simulink model "webserver_start_firstpage_demo"  (Simulink 7.3)
settings: Solver=FixedStepDiscrete  SolverMode=SingleTasking  StartTime=0.0  StopTime=10.0  RelTol=1e-3
PreLoadFcn:
  | waijung.modelPreload; % Required for working with Waijung Blockset. Do not remove.
undefined symbols (not defined in the file): A1, A2, A7, B13, C1, C4, C5, G11, G13, HSEOSC, Link, LQFP144, ST, STM32F429ZI
libraries: waijung_webserver x3, stm32f4_adc_lib x1, stm32f4_io_lib x1, stm32f4_device_config_lib x1
CloseFcn:
  | waijung.modelClose; % Required for working with Waijung Blockset. Do not remove.
settings Model: Creator=Krisada  LastModifiedBy=Krisada
settings OptimizationCC: InlineParams=on  OptimizeModelRefInitCode=on  LifeSpan=1
settings HardwareCC: ProdEndianess=LittleEndian  ProdHWDeviceType=ARM Compatible->Cortex - M4  TargetEndianess=LittleEndian  TargetHWDeviceType=ARM Compatible->Cortex - M4
settings RTWCC: SystemTargetFile=stm32f4.tlc  GenerateMakefile=off  TemplateMakefile=ert_default_tmf  Description=STM32F4 Target  ProcessScript=stm32f4_make_rtw_hook
settings CodeAppCC: IgnoreCustomStorageClasses=off
settings STFCustomTargetCC: ModelReferenceCompliant=off  CombineOutputUpdateFcns=on  ERTCustomFileBanners=on  SupportContinuousTime=off  SupportNonInlinedSFcns=off  SystemTargetFile=stm32f4.tlc
settings ERTTargetCC: MultiwordLength=2048  ModelReferenceCompliant=off  ParMdlRefBuildCompliant=off  CompOptLevelCompliant=off  ERTFirstTimeCompliant=off  ModelStepFunctionPrototypeControlCompliant=off  CPPClassGenCompliant=off  ExtModeMexFile=noextcomm  InlinedParameterPlacement=NonHierarchical  ERTSrcFileBannerTemplate=stm32f4_code_template.cgt  ERTHdrFileBannerTemplate=stm32f4_code_template.cgt  ERTDataSrcFileTemplate=stm32f4_code_template.cgt  ERTDataHdrFileTemplate=stm32f4_code_template.cgt  ERTCustomFileTemplate=stm32f4_file_process.tlc

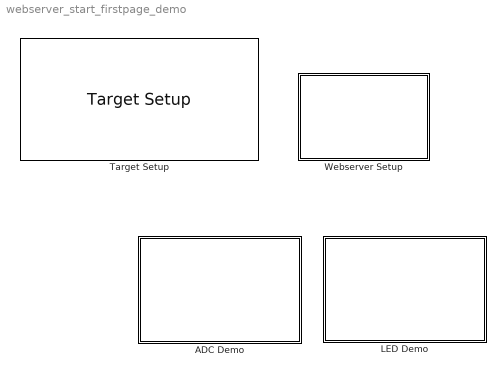
== system webserver_start_firstpage_demo ==
  ADC Demo : Subsystem
  LED Demo : Subsystem
  Target Setup : stm32f4_device_config_lib/Target Setup  Priority=100  compiler=GNU ARM  previous_compiler=GNU ARM  mcu=STM32F429ZI (LQFP144)  mcustr=STM32F429ZI  clockconfig=HSEOSC-8MHz  system_stm32f4xx_c_path=F:\trunk\targets\stm32f4_target\stm32f4\utils\system_stm32f4xx_default\STM32F429_439xx\hseosc8mhz  showmemoryconfiguration=on  stacksize=0x2000  heapsize=0x2000  enableautocompiledownload=on  fullchiperase=on  programmerinterface=ST-Link  editctrlstr=on  compilercontrolstr=$(patsubst %, -I%, .) -mcpu=cortex-m4 -mthumb -mthumb-interwork -mfloat-abi=hard -mfpu=fpv4-sp-d16 -ffast-math -Wall -Wextra -Ofast  assemblercontrolstr=$(patsubst %, -I%, .) -mcpu=cortex-m4 -mthumb -mthumb-interwork -mfloat-abi=hard -mfpu=fpv4-sp-d16 -ffast-math -Wall -Wextra -Ofast -Wa,-amhls=$(<:.s=.lst) -D__STACK_SIZE=$(STACK_SIZE) -D__HEAP_SIZE=$(HEAP_SIZE)  linkercontrolstr=-T$(LD_SCRIPT) -g -Wl,-Map=$(MAP),--cref,--no-warn-mismatch -mcpu=cortex-m4 -mthumb -mthumb-interwork -mfloat-abi=hard -mfpu=fpv4-sp-d16 -specs=nosys.specs  runafterdownload=on  execprofile=None  profileruart=1  profilerbaud=115200  profilertxpin=D8  profilerinitstr=0.01,180000000,1800000,115200,0  manualsetsampletime=off  sampletime=0.01  blockid=TargetSetup  systickreloadvalue=1800000  hseval=8000000  lastprofileruart=1  hclk=180000000  flashorigin=0x8000000  flashlength=2048k  ramorigin=0x20000000  ramlength=192k  useextram=off
  Webserver Setup : Subsystem

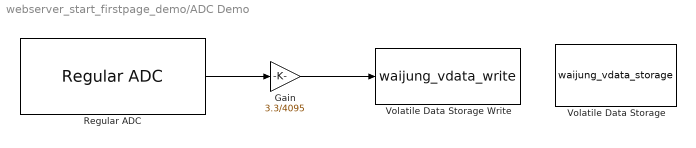
== system webserver_start_firstpage_demo/ADC Demo ==
  Gain : Gain  Gain=3.3/4095  ParameterDataType=fixdt(1, 16)  ParameterScaling=2^0  OutDataType=fixdt(1, 16)  OutScaling=2^0
  Regular ADC : stm32f4_adc_lib/Regular ADC  adcmodule=1  outputdatatype=Single  prescaler=2  prescalerstr=ADC_Prescaler_Div2  chsamplingtime=Auto  chsamplingtimestr=ADC_SampleTime_480Cycles  read_an0=off  read_an1=off  read_an2=off  read_an3=off  read_an4=off  read_an5=off  read_an6=off  read_an7=off  read_an8=off  read_an9=on  read_an10=off  read_an11=off  read_an12=off  read_an13=off  read_an14=off  read_an15=off  read_an16=off  read_an17=off  read_an18=off  pinstr=GPIO_Pin_9  usedpinarray="[0  0  0  0  0  0  0  0  0  1  0  0  0  0  0  0  0  0  0]"  usedportidarray=[1]  usedpinidarray=[1]  usedpinidcount=1  sampletime=-1  blockid=ADCDemoRegularADC  enablecustomportlabel=off  cinputportlabel=0  coutputportlabel=Out1, Out2
  Volatile Data Storage : S-Function  FunctionName=waijung_vdata_storage  Parameters=storagetype,storagename,initval,varname,buffersize,initvalstring,sampletime,sampletimestr,blockid,storagetypestr  EnableBusSupport=off  mask(waijung_vdata_storage){storagetype=single, definevolatile=off, storagename=adc1, initval=0, varname=ADCDemoVolatileDataStorage_adc1, buffersize=64, initvalstring='Initial string', webintegration=ReadOnly, weboutputformat='%f', webcgicallback=(void*)0, laststoragetype=single, sampletime=-1, sampletimestr=0.01, blockid=ADCDemoVolatileDataStorage, storagetypestr=float}
      mask prompts: storagetype "Storage Type"; definevolatile "Define with "volatile" keyword"; storagename "Storage Name (must be a valid variable name)"; initval "Initial value (Apply at Power on Reset only)"; varname "Variable name"; buffersize "Size (bytes)"; initvalstring "Initial value (Apply at Power on Reset only)"; webintegration "Web CGI varget/varset integration"; weboutputformat "Web CGI varget output format"; webcgicallback "Web CGI varset callback"; laststoragetype "Last selected Storage Type"; sampletime "Sample time (sec)"; sampletimestr "Compiled sample time (sec) in string"; storagetypestr "Type string"
      mask help:
      | This block implements a volatile Data Storage.
      |
      | Web CGI varset/varget integratiopn:
      | Enable - In webserver application, allow remote access via http.
      | Disable - Variable is use in local only.
      mask init:
      | waijung_vdata_storage_callback('init');
      mask Help: web(fullfile(waijungdocroot,'Volatile_Data_Storage.htm'))
      mask StyleString: popup(double|single|uint32|int32|uint16|int16|uint8|int8|string),checkbox,edit,edit,edit,edit,edit,popup(Disable|ReadOnly|Write/ Read|ReadOnly with KeyValuePair|Write/ Read with KeyValuePair),edit,edit,popup(double|single|uint32|int32|uint16|int16|uint8|int8|string),edit,edit,edit,edit
      mask CallbackString: waijung_vdata_storage_callback('storagetype');||waijung_vdata_storage_callback('storagename');|waijung_vdata_storage_callback('initval');|waijung_vdata_storage_callback('varname');||waijung_vdata_storage_callback('initvalstring');|waijung_vdata_storage_callback('webintegration');|waijung_vdata_storage_callback('weboutputformat');|||waijung_vdata_storage_callback('sampletime');|waijung_vdata_storage_callback('sampletimestr');|waijung_vdata_storage_callback('blockid');|
      mask Display: text(0.5, 0.5, 'Name: adc1\nType: single','ver','middle','hor','center')
  Volatile Data Storage Write : S-Function  FunctionName=waijung_vdata_write  Parameters=storagename,varname,sampletime,sampletimestr,blockid,storagetype,storagetypestr  EnableBusSupport=off  mask(waijung_vdata_write){storagename=adc1, varname=ADCDemoVolatileDataStorage_adc1, sampletime=-1, sampletimestr=0.01, blockid=ADCDemoVolatileDataStorageWrite, storagetype=single, storagetypestr=float}
      mask prompts: storagename "Storage Name"; varname "Variable name"; sampletime "Sample time (sec)"; sampletimestr "Compiled sample time (sec) in string"; storagetype "Data type"; storagetypestr "Data type string"
      mask help: This block implements write data to a buffer.
      mask init:
      | waijung_vdata_write_callback('init');
      mask Help: web(fullfile(waijungdocroot,'Volatile_Data_Storage_Write.htm'))
      mask StyleString: popup(adc1|led1|led2|led3),edit,edit,edit,edit,edit,edit
      mask CallbackString: waijung_vdata_write_callback('storagename');|waijung_vdata_write_callback('varname');|waijung_vdata_write_callback('sampletime');|waijung_vdata_write_callback('sampletimestr');|waijung_vdata_write_callback('blockid');|waijung_vdata_write_callback('storagetype');|
      mask Display: text(0.95, 0.5, 'Buffer: adc1','ver','middle','hor','right');port_label('input',1,'D1(single)')
  wires:
  Regular ADC/1 -> Gain/1
  Gain/1 -> Volatile Data Storage Write/1

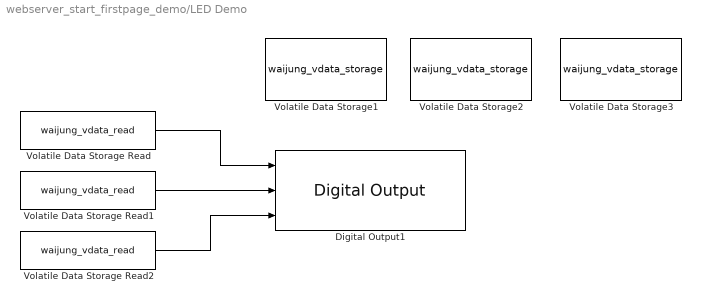
== system webserver_start_firstpage_demo/LED Demo ==
  Digital Output1 : stm32f4_io_lib/Digital Output  use_bitband=on  port=B  speed=100  porttype=Push Pull  porttypestr=PP  use_pin0=on  use_pin1=off  use_pin2=off  use_pin3=off  use_pin4=off  use_pin5=off  use_pin6=off  use_pin7=on  use_pin8=off  use_pin9=off  use_pin10=off  use_pin11=off  use_pin12=off  use_pin13=off  use_pin14=on  use_pin15=off  pinstr=GPIO_Pin_0 | GPIO_Pin_7 | GPIO_Pin_14  usedpinarray="[1  0  0  0  0  0  0  1  0  0  0  0  0  0  1  0]"  bitbandingstr=|  sampletime=-1  sampletimestr=0.01  blockid=LEDDemoDigitalOutput1  enablecustomportlabel=off  globalinit=off  cinputportlabel=In1, In2  coutputportlabel=0
      | #define LEDDemoDigitalOutput1_B0 Peripheral_BB(GPIOB->ODR, 0)  /* Output pin */
      | #define LEDDemoDigitalOutput1_B7 Peripheral_BB(GPIOB->ODR, 7)  /* Output pin */
      | #define LEDDemoDigitalOutput1_B14 Peripheral_BB(GPIOB->ODR, 14)  /* Output pin */
  Volatile Data Storage Read : S-Function  FunctionName=waijung_vdata_read  Parameters=storagename,varname,sampletime,sampletimestr,blockid,storagetype,storagetypestr  EnableBusSupport=off  mask(waijung_vdata_read){storagename=led1, varname=LEDDemoVolatileDataStorage1_led1, sampletime=-1, sampletimestr=0.01, blockid=LEDDemoVolatileDataStorageRead, storagetype=int32, storagetypestr=int32_t}
      mask prompts: storagename "Storage Name"; varname "Variable name"; sampletime "Sample time (sec)"; sampletimestr "Compiled sample time (sec) in string"; storagetype "Data type"; storagetypestr "Data type string"
      mask help: This block implements read data from a buffer.
      mask init:
      | waijung_vdata_read_callback('init');
      mask Help: web(fullfile(waijungdocroot,'Volatile_Data_Storage_Read.htm'))
      mask StyleString: popup(adc1|led1|led2|led3),edit,edit,edit,edit,edit,edit
      mask CallbackString: waijung_vdata_read_callback('storagename');|waijung_vdata_read_callback('varname');|waijung_vdata_read_callback('sampletime');|waijung_vdata_read_callback('sampletimestr');|waijung_vdata_read_callback('blockid');|waijung_vdata_read_callback('storagetype');|
      mask Display: text(0.05, 0.5, 'Buffer: led1','ver','middle','hor','left');port_label('output',1,'D1(int32)')
  Volatile Data Storage Read1 : S-Function  FunctionName=waijung_vdata_read  Parameters=storagename,varname,sampletime,sampletimestr,blockid,storagetype,storagetypestr  EnableBusSupport=off  mask(waijung_vdata_read){storagename=led2, varname=LEDDemoVolatileDataStorage2_led2, sampletime=-1, sampletimestr=0.01, blockid=LEDDemoVolatileDataStorageRead1, storagetype=int32, storagetypestr=int32_t}
      mask prompts: storagename "Storage Name"; varname "Variable name"; sampletime "Sample time (sec)"; sampletimestr "Compiled sample time (sec) in string"; storagetype "Data type"; storagetypestr "Data type string"
      mask help: This block implements read data from a buffer.
      mask init:
      | waijung_vdata_read_callback('init');
      mask Help: web(fullfile(waijungdocroot,'Volatile_Data_Storage_Read.htm'))
      mask StyleString: popup(adc1|led1|led2|led3),edit,edit,edit,edit,edit,edit
      mask CallbackString: waijung_vdata_read_callback('storagename');|waijung_vdata_read_callback('varname');|waijung_vdata_read_callback('sampletime');|waijung_vdata_read_callback('sampletimestr');|waijung_vdata_read_callback('blockid');|waijung_vdata_read_callback('storagetype');|
      mask Display: text(0.05, 0.5, 'Buffer: led2','ver','middle','hor','left');port_label('output',1,'D1(int32)')
  Volatile Data Storage Read2 : S-Function  FunctionName=waijung_vdata_read  Parameters=storagename,varname,sampletime,sampletimestr,blockid,storagetype,storagetypestr  EnableBusSupport=off  mask(waijung_vdata_read){storagename=led3, varname=LEDDemoVolatileDataStorage3_led3, sampletime=-1, sampletimestr=0.01, blockid=LEDDemoVolatileDataStorageRead2, storagetype=int32, storagetypestr=int32_t}
      mask prompts: storagename "Storage Name"; varname "Variable name"; sampletime "Sample time (sec)"; sampletimestr "Compiled sample time (sec) in string"; storagetype "Data type"; storagetypestr "Data type string"
      mask help: This block implements read data from a buffer.
      mask init:
      | waijung_vdata_read_callback('init');
      mask Help: web(fullfile(waijungdocroot,'Volatile_Data_Storage_Read.htm'))
      mask StyleString: popup(adc1|led1|led2|led3),edit,edit,edit,edit,edit,edit
      mask CallbackString: waijung_vdata_read_callback('storagename');|waijung_vdata_read_callback('varname');|waijung_vdata_read_callback('sampletime');|waijung_vdata_read_callback('sampletimestr');|waijung_vdata_read_callback('blockid');|waijung_vdata_read_callback('storagetype');|
      mask Display: text(0.05, 0.5, 'Buffer: led3','ver','middle','hor','left');port_label('output',1,'D1(int32)')
  Volatile Data Storage1 : S-Function  FunctionName=waijung_vdata_storage  Parameters=storagetype,storagename,initval,varname,buffersize,initvalstring,sampletime,sampletimestr,blockid,storagetypestr  EnableBusSupport=off  mask(waijung_vdata_storage){storagetype=int32, definevolatile=off, storagename=led1, initval=0, varname=LEDDemoVolatileDataStorage1_led1, buffersize=64, initvalstring='Initial string', webintegration=Write/ Read, weboutputformat='%d', webcgicallback=(void*)0, laststoragetype=int32, sampletime=-1, sampletimestr=0.01, blockid=LEDDemoVolatileDataStorage1, storagetypestr=int32_t}
      mask prompts: storagetype "Storage Type"; definevolatile "Define with "volatile" keyword"; storagename "Storage Name (must be a valid variable name)"; initval "Initial value (Apply at Power on Reset only)"; varname "Variable name"; buffersize "Size (bytes)"; initvalstring "Initial value (Apply at Power on Reset only)"; webintegration "Web CGI varget/varset integration"; weboutputformat "Web CGI varget output format"; webcgicallback "Web CGI varset callback"; laststoragetype "Last selected Storage Type"; sampletime "Sample time (sec)"; sampletimestr "Compiled sample time (sec) in string"; storagetypestr "Type string"
      mask help:
      | This block implements a volatile Data Storage.
      |
      | Web CGI varset/varget integratiopn:
      | Enable - In webserver application, allow remote access via http.
      | Disable - Variable is use in local only.
      mask init:
      | waijung_vdata_storage_callback('init');
      mask Help: web(fullfile(waijungdocroot,'Volatile_Data_Storage.htm'))
      mask StyleString: popup(double|single|uint32|int32|uint16|int16|uint8|int8|string),checkbox,edit,edit,edit,edit,edit,popup(Disable|ReadOnly|Write/ Read|ReadOnly with KeyValuePair|Write/ Read with KeyValuePair),edit,edit,popup(double|single|uint32|int32|uint16|int16|uint8|int8|string),edit,edit,edit,edit
      mask CallbackString: waijung_vdata_storage_callback('storagetype');||waijung_vdata_storage_callback('storagename');|waijung_vdata_storage_callback('initval');|waijung_vdata_storage_callback('varname');||waijung_vdata_storage_callback('initvalstring');|waijung_vdata_storage_callback('webintegration');|waijung_vdata_storage_callback('weboutputformat');|||waijung_vdata_storage_callback('sampletime');|waijung_vdata_storage_callback('sampletimestr');|waijung_vdata_storage_callback('blockid');|
      mask Display: text(0.5, 0.5, 'Name: led1\nType: int32','ver','middle','hor','center')
  Volatile Data Storage2 : S-Function  FunctionName=waijung_vdata_storage  Parameters=storagetype,storagename,initval,varname,buffersize,initvalstring,sampletime,sampletimestr,blockid,storagetypestr  EnableBusSupport=off  mask(waijung_vdata_storage){storagetype=int32, definevolatile=off, storagename=led2, initval=0, varname=LEDDemoVolatileDataStorage2_led2, buffersize=64, initvalstring='Initial string', webintegration=Write/ Read, weboutputformat='%d', webcgicallback=(void*)0, laststoragetype=int32, sampletime=-1, sampletimestr=0.01, blockid=LEDDemoVolatileDataStorage2, storagetypestr=int32_t}
      mask prompts: storagetype "Storage Type"; definevolatile "Define with "volatile" keyword"; storagename "Storage Name (must be a valid variable name)"; initval "Initial value (Apply at Power on Reset only)"; varname "Variable name"; buffersize "Size (bytes)"; initvalstring "Initial value (Apply at Power on Reset only)"; webintegration "Web CGI varget/varset integration"; weboutputformat "Web CGI varget output format"; webcgicallback "Web CGI varset callback"; laststoragetype "Last selected Storage Type"; sampletime "Sample time (sec)"; sampletimestr "Compiled sample time (sec) in string"; storagetypestr "Type string"
      mask help:
      | This block implements a volatile Data Storage.
      |
      | Web CGI varset/varget integratiopn:
      | Enable - In webserver application, allow remote access via http.
      | Disable - Variable is use in local only.
      mask init:
      | waijung_vdata_storage_callback('init');
      mask Help: web(fullfile(waijungdocroot,'Volatile_Data_Storage.htm'))
      mask StyleString: popup(double|single|uint32|int32|uint16|int16|uint8|int8|string),checkbox,edit,edit,edit,edit,edit,popup(Disable|ReadOnly|Write/ Read|ReadOnly with KeyValuePair|Write/ Read with KeyValuePair),edit,edit,popup(double|single|uint32|int32|uint16|int16|uint8|int8|string),edit,edit,edit,edit
      mask CallbackString: waijung_vdata_storage_callback('storagetype');||waijung_vdata_storage_callback('storagename');|waijung_vdata_storage_callback('initval');|waijung_vdata_storage_callback('varname');||waijung_vdata_storage_callback('initvalstring');|waijung_vdata_storage_callback('webintegration');|waijung_vdata_storage_callback('weboutputformat');|||waijung_vdata_storage_callback('sampletime');|waijung_vdata_storage_callback('sampletimestr');|waijung_vdata_storage_callback('blockid');|
      mask Display: text(0.5, 0.5, 'Name: led2\nType: int32','ver','middle','hor','center')
  Volatile Data Storage3 : S-Function  FunctionName=waijung_vdata_storage  Parameters=storagetype,storagename,initval,varname,buffersize,initvalstring,sampletime,sampletimestr,blockid,storagetypestr  EnableBusSupport=off  mask(waijung_vdata_storage){storagetype=int32, definevolatile=off, storagename=led3, initval=0, varname=LEDDemoVolatileDataStorage3_led3, buffersize=64, initvalstring='Initial string', webintegration=Write/ Read, weboutputformat='%d', webcgicallback=(void*)0, laststoragetype=int32, sampletime=-1, sampletimestr=0.01, blockid=LEDDemoVolatileDataStorage3, storagetypestr=int32_t}
      mask prompts: storagetype "Storage Type"; definevolatile "Define with "volatile" keyword"; storagename "Storage Name (must be a valid variable name)"; initval "Initial value (Apply at Power on Reset only)"; varname "Variable name"; buffersize "Size (bytes)"; initvalstring "Initial value (Apply at Power on Reset only)"; webintegration "Web CGI varget/varset integration"; weboutputformat "Web CGI varget output format"; webcgicallback "Web CGI varset callback"; laststoragetype "Last selected Storage Type"; sampletime "Sample time (sec)"; sampletimestr "Compiled sample time (sec) in string"; storagetypestr "Type string"
      mask help:
      | This block implements a volatile Data Storage.
      |
      | Web CGI varset/varget integratiopn:
      | Enable - In webserver application, allow remote access via http.
      | Disable - Variable is use in local only.
      mask init:
      | waijung_vdata_storage_callback('init');
      mask Help: web(fullfile(waijungdocroot,'Volatile_Data_Storage.htm'))
      mask StyleString: popup(double|single|uint32|int32|uint16|int16|uint8|int8|string),checkbox,edit,edit,edit,edit,edit,popup(Disable|ReadOnly|Write/ Read|ReadOnly with KeyValuePair|Write/ Read with KeyValuePair),edit,edit,popup(double|single|uint32|int32|uint16|int16|uint8|int8|string),edit,edit,edit,edit
      mask CallbackString: waijung_vdata_storage_callback('storagetype');||waijung_vdata_storage_callback('storagename');|waijung_vdata_storage_callback('initval');|waijung_vdata_storage_callback('varname');||waijung_vdata_storage_callback('initvalstring');|waijung_vdata_storage_callback('webintegration');|waijung_vdata_storage_callback('weboutputformat');|||waijung_vdata_storage_callback('sampletime');|waijung_vdata_storage_callback('sampletimestr');|waijung_vdata_storage_callback('blockid');|
      mask Display: text(0.5, 0.5, 'Name: led3\nType: int32','ver','middle','hor','center')
  wires:
  Volatile Data Storage Read/1 -> Digital Output1/1
  Volatile Data Storage Read1/1 -> Digital Output1/2
  Volatile Data Storage Read2/1 -> Digital Output1/3

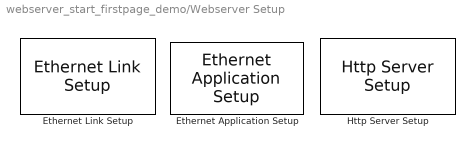
== system webserver_start_firstpage_demo/Webserver Setup ==
  Ethernet Application Setup : waijung_webserver/Ethernet Application Setup  conf=Setup  ipaddress=192.168.1.42  netmask=255.255.255.0  gateway=192.168.1.1  macaddress=02-00-00-00-00-00  dhcp=off  timerscaler=50  portpinstr=0  sampletime=-1  blockid=WebserverSetupEthernetApplicationSetup  inputporttype=[]  inputportwidth=[]  inputportlabel={}  outputporttype=[]  outputportwidth=[]  outputportlabel={}  compat=0  optionstring="[\"Dummy\",\"192\",\"168\",\"1\",\"42\",\"255\",\"255\",\"255\",\"0\",\"192\",\"168\",\"1\",\"1\",\"02\",\"00\",\"00\",\"00\",\"00\",\"00\",\"off\",\"50\"]"
  Ethernet Link Setup : waijung_webserver/Ethernet Link Setup  conf=Setup  interfacepin=Manual  chipaddress=0  wj_interfacetype=RMII  pin_mdio=A2  pin_mdc=C1  pin_pps=Not used  pin_crs=A0  pin_col=A3  pin_dv=A7  pin_rxclk=A1  pin_rxer=B10  pin_rxd0=C4  pin_rxd1=C5  pin_rxd2=B0  pin_rxd3=B1  pin_txclk=C3  pin_txen=G11  pin_txd0=G13  pin_txd1=B13  pin_txd2=C2  pin_txd3=E2  portpinstr=A1,A2,A7,G11,G13,B13,C1,C4,C5,  sampletime=-1  blockid=WebserverSetupEthernetLinkSetup  inputporttype=[]  inputportwidth=[]  inputportlabel={}  outputporttype=[]  outputportwidth=[]  outputportlabel={}  compat=0  optionstring="[\"xxx\",\"on\",\"on\",\"on\",\"off\",\"off\",\"off\",\"on\",\"off\",\"off\",\"off\",\"on\",\"on\",\"off\",\"on\",\"off\",\"off\",\"off\",\"off\",\"off\",\"on\",\"on\",\"on\",\"on\",\"off\",\"off\",\"on\",\"on\",\"A\",\"0\",\"A\",\"1\",\"A\",\"2\",\"A\",\"3\",\"A\",\"7\",\"B\",\"0\",\"B\",\"1\",\"N\",\"ot used\",\"E\",\"2\",\"B\",\"10\",\"G\",\"11\",\"G\",\"13\",\"B\",\"13\",\"C\",\"1\",\"C\",\"2\",\"C\",\"3\",\"C\",\"4\",\"C\",\"5\",\"RMII\",\"0\"]"
  Http Server Setup : waijung_webserver/Http Server Setup  conf=Setup  port=80  ssl=Disable  sqlite=Disable  iap=Disable  mempool=8  debugport=Disable  portpinstr=0  sampletime=-1  blockid=WebserverSetupHttpServerSetup  inputporttype=[]  inputportwidth=[]  inputportlabel={}  outputporttype=[]  outputportwidth=[]  outputportlabel={}  compat=0  optionstring="[\"80\",\"0\",\"0\",\"Disable\",\"Disable\",\"8\",\"17.02b\",\"\",\"\",\"\",\"adc1\",\"single\",\"ADCDemoVolatileDataStorage_adc1\",\"1\",\"0\",\"0\",\"(void*)0\",\"%f\",\"\",\"\",\"led1\",\"int32\",\"LEDDemoVolatileDataStorage1_led1\",\"1\",\"1\",\"0\",\"(void*)0\",\"%d\",\"\",\"\",\"led2\",\"int32\",\"LEDDemoVolatileDataStorage2_led2\",\"1\",\"1\",\"0\",\"(void*)0\",\"%d\",\"\",\"\",\"led3\",\"int32\",\"LEDDemoVolatileDataStorage3_led3\",\"1\",\"1\",\"0\",\"(void*)0\",\"%d\",\"\",\"\"]"
